simulink model "testListenerMdlFinal"  (R2012b)
settings: Solver=FixedStepDiscrete  StartTime=0.0  StopTime=10.0  FixedStep=.1  RelTol=1e-3
PreLoadFcn:
  | myBusDef
StartFcn:
  | % Full path to the block
  | blk = 'testListenerMdl/BusCreator';
  | 
  | % Attach the event listener
  | h = add_exec_event_listener(blk, ...
  |          'PostOutputs', @displayBusdata);
libraries: aerolibanimutils x1
settings Model: BufferReuse=off  Creator=grouleau  LastModifiedBy=grouleau
settings DataIOCC: SaveOutput=off
settings OptimizationCC: BlockReduction=off  ConditionallyExecuteInputs=off  OptimizeBlockIOStorage=off  BufferReuse=off  ExpressionFolding=off  LocalBlockOutputs=off
settings DebuggingCC: ParameterPrecisionLossMsg=none

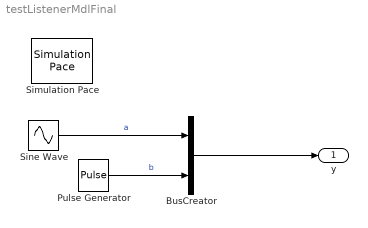
== system testListenerMdlFinal ==
  BusCreator : BusCreator  Inputs=2  OutDataTypeStr=Bus: BO  NonVirtualBus=on
  Pulse Generator : DiscretePulseGenerator  Period=10  PulseWidth=5  SampleTime=.1
  Simulation Pace : aerolibanimutils/Simulation Pace  SimulationPace=1  SleepMode=MATLAB Thread  OutputPaceError=off  SampleTime=.1
      settings: AttributesFormatString=%<SimulationPace> sec/sec
  Sine Wave : Sin  SampleTime=.1
  y : Outport
  wires:
  Sine Wave/1 -> BusCreator/1  "a"
  BusCreator/1 -> y/1
  Pulse Generator/1 -> BusCreator/2  "b"
